simulink model "Autopilot_q_full_5may_new1"  (R2020a)
settings: Solver=ode4  StartTime=0.0  StopTime=300  FixedStep=0.01  RelTol=1e-3
undefined symbols (not defined in the file or in its folder): Aero_cofficients, Atmosphere_pert, Atmospheric_model, Counter_sensor_model, Earth, error_global, flags_global, Guidance_Flags_global, INT_global, param_guidance, Payload_data, Plane_state_mode_finish_catcher_ftr_mode, Plane_state_mode_finish_catcher_fw_mode, Plane_state_mode_finish_catcher_q_mode, Plane_state_mode_finish_catcher_rtr_mode, Plane_state_store, propulsion_model, propulsion_model_int, Structural_data, Thrust_data_store, time_global, WGS84, Wind_data, Wind_model_int, Wind_pert_factor
libraries: simulink x33, aerolibactuator x15, cstblocks x3, aerolibatmos2 x2, aerolibfltsims x1, aerolibtransform2 x1, shared6dof x1
(part 3 of 10)

== system Autopilot_q_full_5may_new1/AUTOPILOT /Autopilot Fixed wing mode/Roll controller ==
  stall_speed : Inport
  Plane_state : Inport  Port=2
  a_y_d : Inport  Port=3
  Aero_coffecients read3 : DataStoreRead  DataStoreName=Aero_cofficients  DataStoreElements=Aero_cofficients(:,:)
  Constant{6..11} (6 alike) : Constant
  Data Store Read : DataStoreRead  DataStoreName=Thrust_data_store  DataStoreElements=Thrust_data_store(:,:)
  Data Store Read1 : DataStoreRead  DataStoreName=param_guidance  DataStoreElements=param_guidance(:)
  Data Store Read13 : DataStoreRead  DataStoreName=propulsion_model  DataStoreElements=propulsion_model(:)
  Data Store Read15 : DataStoreRead  DataStoreName=Atmospheric_model
  Data Store Read2 : DataStoreRead  DataStoreName=Wind_data  DataStoreElements=Wind_data(:)
  Digital Clock : DigitalClock  SampleTime=0.01
  Gain{,1..3} (4 alike) : Gain  Gain=57.3
  MATLAB Function1 : MATLAB Function  TreatAsAtomicUnit=on
  MATLAB Function2 : MATLAB Function  TreatAsAtomicUnit=on
  PID Controller (2DOF) : simulink/Continuous/PID Controller (2DOF)  Controller=PID  Form=Parallel  TimeDomain=Discrete-time  UseExternalTs=off  SampleTime=0.01  IntegratorMethod=Forward Euler  FilterMethod=Forward Euler  ControllerParametersSource=internal  P=4.0  I=0.3  D=0  UseFilter=on  N=100  b=1  c=1  TunerSelectOption=Transfer Function Based (PID Tuner App)  InitialConditionSource=internal  InitialConditionForIntegrator=0  InitialConditionForFilter=0  DifferentiatorICPrevScaledInput=0  ExternalReset=none  TrackingMode=off  Kt=1  LimitOutput=off  UpperSaturationLimit=inf  LowerSaturationLimit=-inf  LinearizeAsGain=on  AntiWindupMode=none  Kb=1  POutMin=[]  POutMax=[]  IOutMin=[]  IOutMax=[]  DOutMin=[]  DOutMax=[]  NOutMin=[]  NOutMax=[]  bOutMin=[]  bOutMax=[]  cOutMin=[]  cOutMax=[]  SumOutMin=[]  SumOutMax=[]  SaturationOutMin=[]  SaturationOutMax=[]  PParamMin=[]  PParamMax=[]  IParamMin=[]  IParamMax=[]  DParamMin=[]  DParamMax=[]  NParamMin=[]  NParamMax=[]  bParamMin=[]  bParamMax=[]  cParamMin=[]  cParamMax=[]  KbParamMin=[]  KbParamMax=[]  KtParamMin=[]  KtParamMax=[]  KbOutMin=[]  KbOutMax=[]  KtOutMin=[]  KtOutMax=[]  IntegratorOutMin=[]  IntegratorOutMax=[]  FilterOutMin=[]  FilterOutMax=[]  SumI1OutMin=[]  SumI1OutMax=[]  SumI2OutMin=[]  SumI2OutMax=[]  SumI3OutMin=[]  SumI3OutMax=[]  SumI4OutMin=[]  SumI4OutMax=[]  SumDOutMin=[]  SumDOutMax=[]  Sum1OutMin=[]  Sum1OutMax=[]  Sum2OutMin=[]  Sum2OutMax=[]  Sum3OutMin=[]  Sum3OutMax=[]  DifferentiatorOutMin=[]  DifferentiatorOutMax=[]  FilterDiffOutCoefMin=[]  FilterDiffOutCoefMax=[]  ReciprocalOutMin=[]  ReciprocalOutMax=[]  SumDenOutMin=[]  SumDenOutMax=[]  SumNumOutMin=[]  SumNumOutMax=[]  DivideOutMin=[]  DivideOutMax=[]  UdiffTsProdOutMin=[]  UdiffTsProdOutMax=[]  NTsProdOutMin=[]  NTsProdOutMax=[]  UintegralTsProdOutMin=[]  UintegralTsProdOutMax=[]  UngainTsProdOutMin=[]  UngainTsProdOutMax=[]  IntegratorContinuousStateAttributes=''  IntegratorStateMustResolveToSignalObject=off  IntegratorRTWStateStorageClass=Auto  FilterContinuousStateAttributes=''  FilterStateMustResolveToSignalObject=off  FilterRTWStateStorageClass=Auto  ParallelPVariant=InternalParameters  IdealPVariant=Disabled  IVariant=InternalParameters  DVariant=InternalParameters  bVariant=InternalParameters  cVariant=InternalParameters  IntegratorVariant=Discrete  SatVariant=Disabled  AWVariant=Passthrough  PCopyVariant=Disabled  TRVariant=Disabled  FdbkBlocksVariant=Forward  IdealPFdbkVariant=Disabled  SatFdbkVariant=Disabled  DerivativeFilterVariant=ForwardEulerFilter  NVariant=InternalParameters  NCopyVariant=Disabled  FilterICVariant=InternalICsFilter  IntegratorICVariant=InternalICs  ExternalResetVariant=Disabled  TRSumVariant=Passthrough  SumFdbkVariant=Disabled  SumVariant=Sum_PID  TsampFilterVariant=InternalTs  TsampNgainVariant=Passthrough  TsampIntegralVariant=Passthrough
  PID Controller (2DOF)1 : simulink/Continuous/PID Controller (2DOF)  Controller=PID  Form=Parallel  TimeDomain=Discrete-time  UseExternalTs=off  SampleTime=0.01  IntegratorMethod=Forward Euler  FilterMethod=Forward Euler  ControllerParametersSource=internal  P=12.0  I=6.0  D=0  UseFilter=on  N=100  b=1  c=1  TunerSelectOption=Transfer Function Based (PID Tuner App)  InitialConditionSource=internal  InitialConditionForIntegrator=0  InitialConditionForFilter=0  DifferentiatorICPrevScaledInput=0  ExternalReset=none  TrackingMode=off  Kt=1  LimitOutput=off  UpperSaturationLimit=inf  LowerSaturationLimit=-inf  LinearizeAsGain=on  AntiWindupMode=none  Kb=1  POutMin=[]  POutMax=[]  IOutMin=[]  IOutMax=[]  DOutMin=[]  DOutMax=[]  NOutMin=[]  NOutMax=[]  bOutMin=[]  bOutMax=[]  cOutMin=[]  cOutMax=[]  SumOutMin=[]  SumOutMax=[]  SaturationOutMin=[]  SaturationOutMax=[]  PParamMin=[]  PParamMax=[]  IParamMin=[]  IParamMax=[]  DParamMin=[]  DParamMax=[]  NParamMin=[]  NParamMax=[]  bParamMin=[]  bParamMax=[]  cParamMin=[]  cParamMax=[]  KbParamMin=[]  KbParamMax=[]  KtParamMin=[]  KtParamMax=[]  KbOutMin=[]  KbOutMax=[]  KtOutMin=[]  KtOutMax=[]  IntegratorOutMin=[]  IntegratorOutMax=[]  FilterOutMin=[]  FilterOutMax=[]  SumI1OutMin=[]  SumI1OutMax=[]  SumI2OutMin=[]  SumI2OutMax=[]  SumI3OutMin=[]  SumI3OutMax=[]  SumI4OutMin=[]  SumI4OutMax=[]  SumDOutMin=[]  SumDOutMax=[]  Sum1OutMin=[]  Sum1OutMax=[]  Sum2OutMin=[]  Sum2OutMax=[]  Sum3OutMin=[]  Sum3OutMax=[]  DifferentiatorOutMin=[]  DifferentiatorOutMax=[]  FilterDiffOutCoefMin=[]  FilterDiffOutCoefMax=[]  ReciprocalOutMin=[]  ReciprocalOutMax=[]  SumDenOutMin=[]  SumDenOutMax=[]  SumNumOutMin=[]  SumNumOutMax=[]  DivideOutMin=[]  DivideOutMax=[]  UdiffTsProdOutMin=[]  UdiffTsProdOutMax=[]  NTsProdOutMin=[]  NTsProdOutMax=[]  UintegralTsProdOutMin=[]  UintegralTsProdOutMax=[]  UngainTsProdOutMin=[]  UngainTsProdOutMax=[]  IntegratorContinuousStateAttributes=''  IntegratorStateMustResolveToSignalObject=off  IntegratorRTWStateStorageClass=Auto  FilterContinuousStateAttributes=''  FilterStateMustResolveToSignalObject=off  FilterRTWStateStorageClass=Auto  ParallelPVariant=InternalParameters  IdealPVariant=Disabled  IVariant=InternalParameters  DVariant=InternalParameters  bVariant=InternalParameters  cVariant=InternalParameters  IntegratorVariant=Discrete  SatVariant=Disabled  AWVariant=Passthrough  PCopyVariant=Disabled  TRVariant=Disabled  FdbkBlocksVariant=Forward  IdealPFdbkVariant=Disabled  SatFdbkVariant=Disabled  DerivativeFilterVariant=ForwardEulerFilter  NVariant=InternalParameters  NCopyVariant=Disabled  FilterICVariant=InternalICsFilter  IntegratorICVariant=InternalICs  ExternalResetVariant=Disabled  TRSumVariant=Passthrough  SumFdbkVariant=Disabled  SumVariant=Sum_PID  TsampFilterVariant=InternalTs  TsampNgainVariant=Passthrough  TsampIntegralVariant=Passthrough
  Scope : Scope  NumInputPorts=2
  Scope1 : Scope  NumInputPorts=2
  Structure_data_read2 : DataStoreRead  DataStoreName=Structural_data  DataStoreElements=Structural_data(:,:)
  Terminator : Terminator
  mass : DataStoreRead  DataStoreName=Structural_data  DataStoreElements=Structural_data(1,1)
  p : DataStoreRead  DataStoreName=Plane_state_store  DataStoreElements=Plane_state_store(1,4)
  phi : DataStoreRead  DataStoreName=Plane_state_store  DataStoreElements=Plane_state_store(1,7)
  pqr,phi,theta,psi : DataStoreRead  DataStoreName=Plane_state_store  DataStoreElements=Plane_state_store(1,4:9)
  p_dot_d : Outport  VectorParamsAs1DForOutWhenUnconnected=off
  wires:
  p/1 -> Gain3/1, PID Controller (2DOF)1/2
  phi/1 -> PID Controller (2DOF)/2, Gain1/1
  pqr,phi,theta,psi/1 -> MATLAB Function2/1(angular_state)
  PID Controller (2DOF)/1 -> MATLAB Function2/2(phi_dot_d)
  mass/1 -> MATLAB Function1/3(mass)
  Data Store Read/1 -> MATLAB Function1/2(Thrust)
  Aero_coffecients read3/1 -> MATLAB Function1/5(aero_data)
  Digital Clock/1 -> MATLAB Function1/1(t)
  Structure_data_read2/1 -> MATLAB Function1/6(structure_data)
  MATLAB Function1/1(phi_d) -> PID Controller (2DOF)/1, Gain/1
  PID Controller (2DOF)1/1 -> p_dot_d/1
  a_y_d/1 -> MATLAB Function1/4(a_y_d)
  Plane_state/1 -> MATLAB Function1/7(Plane_state)
  Gain/1 -> Scope/1
  Gain1/1 -> Scope/2
  Gain2/1 -> Scope1/1
  Gain3/1 -> Scope1/2
  MATLAB Function2/1(p_d) -> Gain2/1, PID Controller (2DOF)1/1
  Data Store Read1/1 -> MATLAB Function1/8(param_guidance)
  stall_speed/1 -> Terminator/1
  Data Store Read2/1 -> MATLAB Function1/9(Wind_ned)
  Data Store Read13/1 -> MATLAB Function1/10(propulsion_data)
  Data Store Read15/1 -> MATLAB Function1/11(atmos_data)
  Constant6/1 -> MATLAB Function1/12(data2)
  Constant7/1 -> MATLAB Function1/13(data3)
  Constant8/1 -> MATLAB Function1/15(data4)
  Constant9/1 -> MATLAB Function1/14(data5)
  Constant10/1 -> MATLAB Function1/16(data6)
  Constant11/1 -> MATLAB Function1/17(data7)

== system Autopilot_q_full_5may_new1/AUTOPILOT /Autopilot Fixed wing mode/Trim setting ==
  "aero " : Inport
  "struct " : Inport  Port=2
  V_trim : Inport  Port=3
  Data Store Read11 : DataStoreRead  DataStoreName=propulsion_model  DataStoreElements=propulsion_model(:)
  Data Store Read14 : DataStoreRead  DataStoreName=Atmospheric_model
  MATLAB Function : MATLAB Function  TreatAsAtomicUnit=on
  alpha_trim : Outport  VectorParamsAs1DForOutWhenUnconnected=off
  beta_trim : Outport  Port=2  VectorParamsAs1DForOutWhenUnconnected=off
  delta_e_trim : Outport  Port=3  VectorParamsAs1DForOutWhenUnconnected=off
  delta_a_trim : Outport  Port=4  VectorParamsAs1DForOutWhenUnconnected=off
  delta_r_trim : Outport  Port=5  VectorParamsAs1DForOutWhenUnconnected=off
  Tx_trim : Outport  Port=6  VectorParamsAs1DForOutWhenUnconnected=off
  stall_speed : Outport  Port=7  VectorParamsAs1DForOutWhenUnconnected=off
  wires:
  "aero "/1 -> MATLAB Function/1(aero_data)
  "struct "/1 -> MATLAB Function/2(structure_data)
  V_trim/1 -> MATLAB Function/3(V_trim)
  MATLAB Function/1(alpha_trim) -> alpha_trim/1
  MATLAB Function/2(beta_trim) -> beta_trim/1
  MATLAB Function/3(delta_e_trim) -> delta_e_trim/1
  MATLAB Function/4(delta_a_trim) -> delta_a_trim/1
  MATLAB Function/5(delta_r_trim) -> delta_r_trim/1
  MATLAB Function/6(Tx_trim) -> Tx_trim/1
  MATLAB Function/7(stall_speed) -> stall_speed/1
  Data Store Read11/1 -> MATLAB Function/4(propulsion_data)
  Data Store Read14/1 -> MATLAB Function/5(atmos_data)

== system Autopilot_q_full_5may_new1/AUTOPILOT /Autopilot Fixed wing mode/beta controller ==
  acc_d : Inport
  Plane_state : Inport  Port=2
  stall_speed : Inport  Port=3
  Aero_coffecients read2 : DataStoreRead  DataStoreName=Aero_cofficients  DataStoreElements=Aero_cofficients(:,:)
  Constant{6..11} (6 alike) : Constant
  Data Store Read : DataStoreRead  DataStoreName=Wind_data  DataStoreElements=Wind_data(:)
  Data Store Read13 : DataStoreRead  DataStoreName=propulsion_model  DataStoreElements=propulsion_model(:)
  Data Store Read15 : DataStoreRead  DataStoreName=Atmospheric_model
  Data Store Read3 : DataStoreRead  DataStoreName=Thrust_data_store  DataStoreElements=Thrust_data_store(:,:)
  Gain{,1..3} (4 alike) : Gain  Gain=57.3
  PID Controller (2DOF)1 : simulink/Continuous/PID Controller (2DOF)  Controller=PID  TimeDomain=Discrete-time  SampleTime=0.01  IntegratorMethod=Forward Euler  FilterMethod=Forward Euler  Form=Parallel  UseFilter=on  ControllerParametersSource=internal  P=1.8  I=0.5  D=0  N=100  b=1  c=1  InitialConditionSource=internal  InitialConditionForIntegrator=0  InitialConditionForFilter=0  ExternalReset=none  LimitOutput=off  UpperSaturationLimit=inf  LowerSaturationLimit=-inf  LinearizeAsGain=on  AntiWindupMode=none  Kb=1  TrackingMode=off  Kt=1  PParamMin=[]  PParamMax=[]  IParamMin=[]  IParamMax=[]  DParamMin=[]  DParamMax=[]  NParamMin=[]  NParamMax=[]  bParamMin=[]  bParamMax=[]  cParamMin=[]  cParamMax=[]  KbParamMin=[]  KbParamMax=[]  KtParamMin=[]  KtParamMax=[]  POutMin=[]  POutMax=[]  IOutMin=[]  IOutMax=[]  DOutMin=[]  DOutMax=[]  NOutMin=[]  NOutMax=[]  bOutMin=[]  bOutMax=[]  cOutMin=[]  cOutMax=[]  KbOutMin=[]  KbOutMax=[]  KtOutMin=[]  KtOutMax=[]  IntegratorOutMin=[]  IntegratorOutMax=[]  FilterOutMin=[]  FilterOutMax=[]  SumOutMin=[]  SumOutMax=[]  Sum1OutMin=[]  Sum1OutMax=[]  Sum2OutMin=[]  Sum2OutMax=[]  Sum3OutMin=[]  Sum3OutMax=[]  SumI1OutMin=[]  SumI1OutMax=[]  SumI2OutMin=[]  SumI2OutMax=[]  SumI3OutMin=[]  SumI3OutMax=[]  SumDOutMin=[]  SumDOutMax=[]  SaturationOutMin=[]  SaturationOutMax=[]  IntegratorContinuousStateAttributes=''  IntegratorStateMustResolveToSignalObject=off  IntegratorRTWStateStorageClass=Auto  FilterContinuousStateAttributes=''  FilterStateMustResolveToSignalObject=off  FilterRTWStateStorageClass=Auto  DifferentiatorICPrevScaledInput=0  DifferentiatorOutMin=[]  DifferentiatorOutMax=[]  FilterDiffOutCoefMin=[]  FilterDiffOutCoefMax=[]  SumDenOutMin=[]  SumDenOutMax=[]  SumNumOutMin=[]  SumNumOutMax=[]  ReciprocalOutMin=[]  ReciprocalOutMax=[]  DivideOutMin=[]  DivideOutMax=[]  TunerSelectOption=Transfer Function Based (PID Tuner App)
  PID Controller (2DOF)2 : simulink/Continuous/PID Controller (2DOF)  Controller=PID  TimeDomain=Discrete-time  SampleTime=0.01  IntegratorMethod=Forward Euler  FilterMethod=Forward Euler  Form=Parallel  UseFilter=on  ControllerParametersSource=internal  P=0.66  I=0  D=0  N=100  b=1  c=1  InitialConditionSource=internal  InitialConditionForIntegrator=0  InitialConditionForFilter=0  ExternalReset=none  LimitOutput=off  UpperSaturationLimit=inf  LowerSaturationLimit=-inf  LinearizeAsGain=on  AntiWindupMode=none  Kb=1  TrackingMode=off  Kt=1  PParamMin=[]  PParamMax=[]  IParamMin=[]  IParamMax=[]  DParamMin=[]  DParamMax=[]  NParamMin=[]  NParamMax=[]  bParamMin=[]  bParamMax=[]  cParamMin=[]  cParamMax=[]  KbParamMin=[]  KbParamMax=[]  KtParamMin=[]  KtParamMax=[]  POutMin=[]  POutMax=[]  IOutMin=[]  IOutMax=[]  DOutMin=[]  DOutMax=[]  NOutMin=[]  NOutMax=[]  bOutMin=[]  bOutMax=[]  cOutMin=[]  cOutMax=[]  KbOutMin=[]  KbOutMax=[]  KtOutMin=[]  KtOutMax=[]  IntegratorOutMin=[]  IntegratorOutMax=[]  FilterOutMin=[]  FilterOutMax=[]  SumOutMin=[]  SumOutMax=[]  Sum1OutMin=[]  Sum1OutMax=[]  Sum2OutMin=[]  Sum2OutMax=[]  Sum3OutMin=[]  Sum3OutMax=[]  SumI1OutMin=[]  SumI1OutMax=[]  SumI2OutMin=[]  SumI2OutMax=[]  SumI3OutMin=[]  SumI3OutMax=[]  SumDOutMin=[]  SumDOutMax=[]  SaturationOutMin=[]  SaturationOutMax=[]  IntegratorContinuousStateAttributes=''  IntegratorStateMustResolveToSignalObject=off  IntegratorRTWStateStorageClass=Auto  FilterContinuousStateAttributes=''  FilterStateMustResolveToSignalObject=off  FilterRTWStateStorageClass=Auto  DifferentiatorICPrevScaledInput=0  DifferentiatorOutMin=[]  DifferentiatorOutMax=[]  FilterDiffOutCoefMin=[]  FilterDiffOutCoefMax=[]  SumDenOutMin=[]  SumDenOutMax=[]  SumNumOutMin=[]  SumNumOutMax=[]  ReciprocalOutMin=[]  ReciprocalOutMax=[]  DivideOutMin=[]  DivideOutMax=[]  TunerSelectOption=Transfer Function Based (PID Tuner App)
  Scope : Scope  NumInputPorts=2
  Scope1 : Scope  NumInputPorts=2
  Structure_data_read1 : DataStoreRead  DataStoreName=Structural_data  DataStoreElements=Structural_data(:,:)
  beta_controller : MATLAB Function  TreatAsAtomicUnit=on
  r_dot_d : Outport  VectorParamsAs1DForOutWhenUnconnected=off
  wires:
  Aero_coffecients read2/1 -> beta_controller/3(aero_data)
  Structure_data_read1/1 -> beta_controller/4(structure_data)
  Data Store Read3/1 -> beta_controller/5(Thrust)
  beta_controller/1(beta_d) -> Gain/1, PID Controller (2DOF)2/1
  Plane_state/1 -> beta_controller/2(Plane_state)
  acc_d/1 -> beta_controller/1(acc_d)
  beta_controller/2(beta) -> PID Controller (2DOF)2/2, Gain1/1
  PID Controller (2DOF)1/1 -> r_dot_d/1
  stall_speed/1 -> beta_controller/6(V_stall)
  Gain/1 -> Scope/1
  Gain1/1 -> Scope/2
  Gain2/1 -> Scope1/1
  beta_controller/3(r) -> PID Controller (2DOF)1/2, Gain3/1
  Gain3/1 -> Scope1/2
  PID Controller (2DOF)2/1 -> Gain2/1, PID Controller (2DOF)1/1
  Data Store Read/1 -> beta_controller/7(Wind_ned)
  Data Store Read13/1 -> beta_controller/8(propulsion_data)
  Data Store Read15/1 -> beta_controller/9(atmos_data)
  Constant6/1 -> beta_controller/10(data2)
  Constant7/1 -> beta_controller/11(data3)
  Constant8/1 -> beta_controller/12(data4)
  Constant9/1 -> beta_controller/13(data5)
  Constant10/1 -> beta_controller/14(data6)
  Constant11/1 -> beta_controller/15(data7)

== system Autopilot_q_full_5may_new1/AUTOPILOT /Autopilot Quad mode/Heading Controller ==
  Data Store Read4 : DataStoreRead  DataStoreName=Plane_state_mode_finish_catcher_rtr_mode  SampleTime=0.01  DataStoreElements=Plane_state_mode_finish_catcher_rtr_mode(9)
  Demux1 : Demux  Outputs=2
  Digital Clock : DigitalClock  SampleTime=0.01
  MATLAB Function : MATLAB Function  TreatAsAtomicUnit=on
  MATLAB Function5 : MATLAB Function  TreatAsAtomicUnit=on
  MATLAB Function6 : MATLAB Function  TreatAsAtomicUnit=on
  PID Controller : simulink/Continuous/PID Controller  Controller=PID  Form=Parallel  TimeDomain=Discrete-time  UseExternalTs=off  SampleTime=0.01  IntegratorMethod=Forward Euler  FilterMethod=Forward Euler  ControllerParametersSource=internal  P=0.66  I=0  D=0  UseFilter=on  N=100  TunerSelectOption=Transfer Function Based (PID Tuner App)  InitialConditionSource=internal  InitialConditionForIntegrator=0  InitialConditionForFilter=0  DifferentiatorICPrevScaledInput=0  ExternalReset=none  TrackingMode=off  Kt=1  LimitOutput=off  UpperSaturationLimit=inf  LowerSaturationLimit=-inf  LinearizeAsGain=on  AntiWindupMode=none  Kb=1  POutMin=[]  POutMax=[]  IOutMin=[]  IOutMax=[]  DOutMin=[]  DOutMax=[]  NOutMin=[]  NOutMax=[]  SumOutMin=[]  SumOutMax=[]  SaturationOutMin=[]  SaturationOutMax=[]  PParamMin=[]  PParamMax=[]  IParamMin=[]  IParamMax=[]  DParamMin=[]  DParamMax=[]  NParamMin=[]  NParamMax=[]  KbParamMin=[]  KbParamMax=[]  KtParamMin=[]  KtParamMax=[]  KbOutMin=[]  KbOutMax=[]  KtOutMin=[]  KtOutMax=[]  IntegratorOutMin=[]  IntegratorOutMax=[]  FilterOutMin=[]  FilterOutMax=[]  SumI1OutMin=[]  SumI1OutMax=[]  SumI2OutMin=[]  SumI2OutMax=[]  SumI3OutMin=[]  SumI3OutMax=[]  SumI4OutMin=[]  SumI4OutMax=[]  SumDOutMin=[]  SumDOutMax=[]  DifferentiatorOutMin=[]  DifferentiatorOutMax=[]  FilterDiffOutCoefMin=[]  FilterDiffOutCoefMax=[]  ReciprocalOutMin=[]  ReciprocalOutMax=[]  SumDenOutMin=[]  SumDenOutMax=[]  SumNumOutMin=[]  SumNumOutMax=[]  DivideOutMin=[]  DivideOutMax=[]  UdiffTsProdOutMin=[]  UdiffTsProdOutMax=[]  NTsProdOutMin=[]  NTsProdOutMax=[]  UintegralTsProdOutMin=[]  UintegralTsProdOutMax=[]  UngainTsProdOutMin=[]  UngainTsProdOutMax=[]  IntegratorContinuousStateAttributes=''  IntegratorStateMustResolveToSignalObject=off  IntegratorRTWStateStorageClass=Auto  FilterContinuousStateAttributes=''  FilterStateMustResolveToSignalObject=off  FilterRTWStateStorageClass=Auto  ParallelPVariant=InternalParameters  IdealPVariant=Disabled  IVariant=InternalParameters  DVariant=InternalParameters  IntegratorVariant=Discrete  SatVariant=Disabled  AWVariant=Passthrough  PCopyVariant=Disabled  TRVariant=Disabled  FdbkBlocksVariant=Forward  IdealPFdbkVariant=Disabled  SatFdbkVariant=Disabled  DerivativeFilterVariant=ForwardEulerFilter  NVariant=InternalParameters  NCopyVariant=Disabled  FilterICVariant=InternalICsFilter  IntegratorICVariant=InternalICs  ExternalResetVariant=Disabled  TRSumVariant=Passthrough  SumFdbkVariant=Disabled  SumVariant=Sum_PID  TsampFilterVariant=InternalTs  TsampNgainVariant=Passthrough  TsampIntegralVariant=Passthrough
  PID Controller (2DOF)5 : simulink/Continuous/PID Controller (2DOF)  Controller=PID  Form=Parallel  TimeDomain=Discrete-time  UseExternalTs=off  SampleTime=0.01  IntegratorMethod=Forward Euler  FilterMethod=Forward Euler  ControllerParametersSource=internal  P=2  I=0.5  D=0  UseFilter=on  N=100  b=1  c=1  TunerSelectOption=Transfer Function Based (PID Tuner App)  InitialConditionSource=internal  InitialConditionForIntegrator=0  InitialConditionForFilter=0  DifferentiatorICPrevScaledInput=0  ExternalReset=none  TrackingMode=off  Kt=1  LimitOutput=off  UpperSaturationLimit=inf  LowerSaturationLimit=-inf  LinearizeAsGain=on  AntiWindupMode=none  Kb=1  POutMin=[]  POutMax=[]  IOutMin=[]  IOutMax=[]  DOutMin=[]  DOutMax=[]  NOutMin=[]  NOutMax=[]  bOutMin=[]  bOutMax=[]  cOutMin=[]  cOutMax=[]  SumOutMin=[]  SumOutMax=[]  SaturationOutMin=[]  SaturationOutMax=[]  PParamMin=[]  PParamMax=[]  IParamMin=[]  IParamMax=[]  DParamMin=[]  DParamMax=[]  NParamMin=[]  NParamMax=[]  bParamMin=[]  bParamMax=[]  cParamMin=[]  cParamMax=[]  KbParamMin=[]  KbParamMax=[]  KtParamMin=[]  KtParamMax=[]  KbOutMin=[]  KbOutMax=[]  KtOutMin=[]  KtOutMax=[]  IntegratorOutMin=[]  IntegratorOutMax=[]  FilterOutMin=[]  FilterOutMax=[]  SumI1OutMin=[]  SumI1OutMax=[]  SumI2OutMin=[]  SumI2OutMax=[]  SumI3OutMin=[]  SumI3OutMax=[]  SumI4OutMin=[]  SumI4OutMax=[]  SumDOutMin=[]  SumDOutMax=[]  Sum1OutMin=[]  Sum1OutMax=[]  Sum2OutMin=[]  Sum2OutMax=[]  Sum3OutMin=[]  Sum3OutMax=[]  DifferentiatorOutMin=[]  DifferentiatorOutMax=[]  FilterDiffOutCoefMin=[]  FilterDiffOutCoefMax=[]  ReciprocalOutMin=[]  ReciprocalOutMax=[]  SumDenOutMin=[]  SumDenOutMax=[]  SumNumOutMin=[]  SumNumOutMax=[]  DivideOutMin=[]  DivideOutMax=[]  UdiffTsProdOutMin=[]  UdiffTsProdOutMax=[]  NTsProdOutMin=[]  NTsProdOutMax=[]  UintegralTsProdOutMin=[]  UintegralTsProdOutMax=[]  UngainTsProdOutMin=[]  UngainTsProdOutMax=[]  IntegratorContinuousStateAttributes=''  IntegratorStateMustResolveToSignalObject=off  IntegratorRTWStateStorageClass=Auto  FilterContinuousStateAttributes=''  FilterStateMustResolveToSignalObject=off  FilterRTWStateStorageClass=Auto  ParallelPVariant=InternalParameters  IdealPVariant=Disabled  IVariant=InternalParameters  DVariant=InternalParameters  bVariant=InternalParameters  cVariant=InternalParameters  IntegratorVariant=Discrete  SatVariant=Disabled  AWVariant=Passthrough  PCopyVariant=Disabled  TRVariant=Disabled  FdbkBlocksVariant=Forward  IdealPFdbkVariant=Disabled  SatFdbkVariant=Disabled  DerivativeFilterVariant=ForwardEulerFilter  NVariant=InternalParameters  NCopyVariant=Disabled  FilterICVariant=InternalICsFilter  IntegratorICVariant=InternalICs  ExternalResetVariant=Disabled  TRSumVariant=Passthrough  SumFdbkVariant=Disabled  SumVariant=Sum_PID  TsampFilterVariant=InternalTs  TsampNgainVariant=Passthrough  TsampIntegralVariant=Passthrough
  p,q,r,phi,theta,psi : DataStoreRead  DataStoreName=Plane_state_store  DataStoreElements=Plane_state_store(1,4:9)
  psi : DataStoreRead  DataStoreName=Plane_state_store  DataStoreElements=Plane_state_store(1,9)
  r : DataStoreRead  DataStoreName=Plane_state_store  DataStoreElements=Plane_state_store(1,6)
  u,v : DataStoreRead  DataStoreName=Plane_state_store  SampleTime=0.01  DataStoreElements=Plane_state_store(1,1:2)
  Out1 : Outport  VectorParamsAs1DForOutWhenUnconnected=off
  wires:
  MATLAB Function5/1(psi_d) -> MATLAB Function/1(psi_d)
  u,v/1 -> Demux1/1
  Data Store Read4/1 -> MATLAB Function5/4("psi_d ")
  Digital Clock/1 -> MATLAB Function5/1(t)
  Demux1/1 -> MATLAB Function5/2(u)
  p,q,r,phi,theta,psi/1 -> MATLAB Function6/1(angular_state)
  psi/1 -> MATLAB Function/2(psi)
  MATLAB Function6/1(r_d) -> PID Controller (2DOF)5/1
  PID Controller/1 -> MATLAB Function6/2(psi_dot_d)
  MATLAB Function/1(psi_error) -> PID Controller/1
  Demux1/2 -> MATLAB Function5/3(v)
  PID Controller (2DOF)5/1 -> Out1/1
  r/1 -> PID Controller (2DOF)5/2

== system Autopilot_q_full_5may_new1/AUTOPILOT /Autopilot Quad mode/Pitch Controller ==
  a_x_d : Inport
  Data Store Read1 : DataStoreRead  DataStoreName=Thrust_data_store
  Digital Clock : DigitalClock  SampleTime=0.01
  MATLAB Function3 : MATLAB Function  TreatAsAtomicUnit=on
  MATLAB Function4 : MATLAB Function  TreatAsAtomicUnit=on
  PID Controller (2DOF)2 : simulink/Continuous/PID Controller (2DOF)  Controller=PID  Form=Parallel  TimeDomain=Discrete-time  UseExternalTs=off  SampleTime=0.01  IntegratorMethod=Forward Euler  FilterMethod=Forward Euler  ControllerParametersSource=internal  P=4.0  I=0  D=0  UseFilter=on  N=100  b=1  c=1  TunerSelectOption=Transfer Function Based (PID Tuner App)  InitialConditionSource=internal  InitialConditionForIntegrator=0  InitialConditionForFilter=0  DifferentiatorICPrevScaledInput=0  ExternalReset=none  TrackingMode=off  Kt=1  LimitOutput=off  UpperSaturationLimit=inf  LowerSaturationLimit=-inf  LinearizeAsGain=on  AntiWindupMode=none  Kb=1  POutMin=[]  POutMax=[]  IOutMin=[]  IOutMax=[]  DOutMin=[]  DOutMax=[]  NOutMin=[]  NOutMax=[]  bOutMin=[]  bOutMax=[]  cOutMin=[]  cOutMax=[]  SumOutMin=[]  SumOutMax=[]  SaturationOutMin=[]  SaturationOutMax=[]  PParamMin=[]  PParamMax=[]  IParamMin=[]  IParamMax=[]  DParamMin=[]  DParamMax=[]  NParamMin=[]  NParamMax=[]  bParamMin=[]  bParamMax=[]  cParamMin=[]  cParamMax=[]  KbParamMin=[]  KbParamMax=[]  KtParamMin=[]  KtParamMax=[]  KbOutMin=[]  KbOutMax=[]  KtOutMin=[]  KtOutMax=[]  IntegratorOutMin=[]  IntegratorOutMax=[]  FilterOutMin=[]  FilterOutMax=[]  SumI1OutMin=[]  SumI1OutMax=[]  SumI2OutMin=[]  SumI2OutMax=[]  SumI3OutMin=[]  SumI3OutMax=[]  SumI4OutMin=[]  SumI4OutMax=[]  SumDOutMin=[]  SumDOutMax=[]  Sum1OutMin=[]  Sum1OutMax=[]  Sum2OutMin=[]  Sum2OutMax=[]  Sum3OutMin=[]  Sum3OutMax=[]  DifferentiatorOutMin=[]  DifferentiatorOutMax=[]  FilterDiffOutCoefMin=[]  FilterDiffOutCoefMax=[]  ReciprocalOutMin=[]  ReciprocalOutMax=[]  SumDenOutMin=[]  SumDenOutMax=[]  SumNumOutMin=[]  SumNumOutMax=[]  DivideOutMin=[]  DivideOutMax=[]  UdiffTsProdOutMin=[]  UdiffTsProdOutMax=[]  NTsProdOutMin=[]  NTsProdOutMax=[]  UintegralTsProdOutMin=[]  UintegralTsProdOutMax=[]  UngainTsProdOutMin=[]  UngainTsProdOutMax=[]  IntegratorContinuousStateAttributes=''  IntegratorStateMustResolveToSignalObject=off  IntegratorRTWStateStorageClass=Auto  FilterContinuousStateAttributes=''  FilterStateMustResolveToSignalObject=off  FilterRTWStateStorageClass=Auto  ParallelPVariant=InternalParameters  IdealPVariant=Disabled  IVariant=InternalParameters  DVariant=InternalParameters  bVariant=InternalParameters  cVariant=InternalParameters  IntegratorVariant=Discrete  SatVariant=Disabled  AWVariant=Passthrough  PCopyVariant=Disabled  TRVariant=Disabled  FdbkBlocksVariant=Forward  IdealPFdbkVariant=Disabled  SatFdbkVariant=Disabled  DerivativeFilterVariant=ForwardEulerFilter  NVariant=InternalParameters  NCopyVariant=Disabled  FilterICVariant=InternalICsFilter  IntegratorICVariant=InternalICs  ExternalResetVariant=Disabled  TRSumVariant=Passthrough  SumFdbkVariant=Disabled  SumVariant=Sum_PID  TsampFilterVariant=InternalTs  TsampNgainVariant=Passthrough  TsampIntegralVariant=Passthrough
  PID Controller (2DOF)3 : simulink/Continuous/PID Controller (2DOF)  Controller=PID  Form=Parallel  TimeDomain=Discrete-time  UseExternalTs=off  SampleTime=0.01  IntegratorMethod=Forward Euler  FilterMethod=Forward Euler  ControllerParametersSource=internal  P=12.0  I=0.1  D=0  UseFilter=on  N=100  b=1  c=1  TunerSelectOption=Transfer Function Based (PID Tuner App)  InitialConditionSource=internal  InitialConditionForIntegrator=0  InitialConditionForFilter=0  DifferentiatorICPrevScaledInput=0  ExternalReset=none  TrackingMode=off  Kt=1  LimitOutput=off  UpperSaturationLimit=inf  LowerSaturationLimit=-inf  LinearizeAsGain=on  AntiWindupMode=none  Kb=1  POutMin=[]  POutMax=[]  IOutMin=[]  IOutMax=[]  DOutMin=[]  DOutMax=[]  NOutMin=[]  NOutMax=[]  bOutMin=[]  bOutMax=[]  cOutMin=[]  cOutMax=[]  SumOutMin=[]  SumOutMax=[]  SaturationOutMin=[]  SaturationOutMax=[]  PParamMin=[]  PParamMax=[]  IParamMin=[]  IParamMax=[]  DParamMin=[]  DParamMax=[]  NParamMin=[]  NParamMax=[]  bParamMin=[]  bParamMax=[]  cParamMin=[]  cParamMax=[]  KbParamMin=[]  KbParamMax=[]  KtParamMin=[]  KtParamMax=[]  KbOutMin=[]  KbOutMax=[]  KtOutMin=[]  KtOutMax=[]  IntegratorOutMin=[]  IntegratorOutMax=[]  FilterOutMin=[]  FilterOutMax=[]  SumI1OutMin=[]  SumI1OutMax=[]  SumI2OutMin=[]  SumI2OutMax=[]  SumI3OutMin=[]  SumI3OutMax=[]  SumI4OutMin=[]  SumI4OutMax=[]  SumDOutMin=[]  SumDOutMax=[]  Sum1OutMin=[]  Sum1OutMax=[]  Sum2OutMin=[]  Sum2OutMax=[]  Sum3OutMin=[]  Sum3OutMax=[]  DifferentiatorOutMin=[]  DifferentiatorOutMax=[]  FilterDiffOutCoefMin=[]  FilterDiffOutCoefMax=[]  ReciprocalOutMin=[]  ReciprocalOutMax=[]  SumDenOutMin=[]  SumDenOutMax=[]  SumNumOutMin=[]  SumNumOutMax=[]  DivideOutMin=[]  DivideOutMax=[]  UdiffTsProdOutMin=[]  UdiffTsProdOutMax=[]  NTsProdOutMin=[]  NTsProdOutMax=[]  UintegralTsProdOutMin=[]  UintegralTsProdOutMax=[]  UngainTsProdOutMin=[]  UngainTsProdOutMax=[]  IntegratorContinuousStateAttributes=''  IntegratorStateMustResolveToSignalObject=off  IntegratorRTWStateStorageClass=Auto  FilterContinuousStateAttributes=''  FilterStateMustResolveToSignalObject=off  FilterRTWStateStorageClass=Auto  ParallelPVariant=InternalParameters  IdealPVariant=Disabled  IVariant=InternalParameters  DVariant=InternalParameters  bVariant=InternalParameters  cVariant=InternalParameters  IntegratorVariant=Discrete  SatVariant=Disabled  AWVariant=Passthrough  PCopyVariant=Disabled  TRVariant=Disabled  FdbkBlocksVariant=Forward  IdealPFdbkVariant=Disabled  SatFdbkVariant=Disabled  DerivativeFilterVariant=ForwardEulerFilter  NVariant=InternalParameters  NCopyVariant=Disabled  FilterICVariant=InternalICsFilter  IntegratorICVariant=InternalICs  ExternalResetVariant=Disabled  TRSumVariant=Passthrough  SumFdbkVariant=Disabled  SumVariant=Sum_PID  TsampFilterVariant=InternalTs  TsampNgainVariant=Passthrough  TsampIntegralVariant=Passthrough
  mass1 : DataStoreRead  DataStoreName=Structural_data  DataStoreElements=Structural_data(1,1)
  p,q,r,phi,theta,psi : DataStoreRead  DataStoreName=Plane_state_store  DataStoreElements=Plane_state_store(1,4:9)
  "q " : DataStoreRead  DataStoreName=Plane_state_store  DataStoreElements=Plane_state_store(1,5)
  theta : DataStoreRead  DataStoreName=Plane_state_store  DataStoreElements=Plane_state_store(1,8)
  Out1 : Outport  VectorParamsAs1DForOutWhenUnconnected=off
  wires:
  "q "/1 -> PID Controller (2DOF)3/2
  Digital Clock/1 -> MATLAB Function3/1(t)
  Data Store Read1/1 -> MATLAB Function3/2(TT)
  PID Controller (2DOF)2/1 -> MATLAB Function4/2(theta_dot_d)
  MATLAB Function4/1(q_d) -> PID Controller (2DOF)3/1
  p,q,r,phi,theta,psi/1 -> MATLAB Function4/1(angular_state)
  theta/1 -> PID Controller (2DOF)2/2
  MATLAB Function3/1(theta_d) -> PID Controller (2DOF)2/1
  mass1/1 -> MATLAB Function3/3(mass)
  a_x_d/1 -> MATLAB Function3/4(a_x_d)
  PID Controller (2DOF)3/1 -> Out1/1

== system Autopilot_q_full_5may_new1/AUTOPILOT /Autopilot Quad mode/Roll Controller ==
  a_y_d : Inport
  Data Store Read : DataStoreRead  DataStoreName=Thrust_data_store
  Digital Clock : DigitalClock  SampleTime=0.01
  MATLAB Function1 : MATLAB Function  TreatAsAtomicUnit=on
  MATLAB Function2 : MATLAB Function  TreatAsAtomicUnit=on
  PID Controller (2DOF) : simulink/Continuous/PID Controller (2DOF)  Controller=PID  Form=Parallel  TimeDomain=Discrete-time  UseExternalTs=off  SampleTime=0.01  IntegratorMethod=Forward Euler  FilterMethod=Forward Euler  ControllerParametersSource=internal  P=4.0  I=0  D=0  UseFilter=on  N=100  b=1  c=1  TunerSelectOption=Transfer Function Based (PID Tuner App)  InitialConditionSource=internal  InitialConditionForIntegrator=0  InitialConditionForFilter=0  DifferentiatorICPrevScaledInput=0  ExternalReset=none  TrackingMode=off  Kt=1  LimitOutput=off  UpperSaturationLimit=inf  LowerSaturationLimit=-inf  LinearizeAsGain=on  AntiWindupMode=none  Kb=1  POutMin=[]  POutMax=[]  IOutMin=[]  IOutMax=[]  DOutMin=[]  DOutMax=[]  NOutMin=[]  NOutMax=[]  bOutMin=[]  bOutMax=[]  cOutMin=[]  cOutMax=[]  SumOutMin=[]  SumOutMax=[]  SaturationOutMin=[]  SaturationOutMax=[]  PParamMin=[]  PParamMax=[]  IParamMin=[]  IParamMax=[]  DParamMin=[]  DParamMax=[]  NParamMin=[]  NParamMax=[]  bParamMin=[]  bParamMax=[]  cParamMin=[]  cParamMax=[]  KbParamMin=[]  KbParamMax=[]  KtParamMin=[]  KtParamMax=[]  KbOutMin=[]  KbOutMax=[]  KtOutMin=[]  KtOutMax=[]  IntegratorOutMin=[]  IntegratorOutMax=[]  FilterOutMin=[]  FilterOutMax=[]  SumI1OutMin=[]  SumI1OutMax=[]  SumI2OutMin=[]  SumI2OutMax=[]  SumI3OutMin=[]  SumI3OutMax=[]  SumI4OutMin=[]  SumI4OutMax=[]  SumDOutMin=[]  SumDOutMax=[]  Sum1OutMin=[]  Sum1OutMax=[]  Sum2OutMin=[]  Sum2OutMax=[]  Sum3OutMin=[]  Sum3OutMax=[]  DifferentiatorOutMin=[]  DifferentiatorOutMax=[]  FilterDiffOutCoefMin=[]  FilterDiffOutCoefMax=[]  ReciprocalOutMin=[]  ReciprocalOutMax=[]  SumDenOutMin=[]  SumDenOutMax=[]  SumNumOutMin=[]  SumNumOutMax=[]  DivideOutMin=[]  DivideOutMax=[]  UdiffTsProdOutMin=[]  UdiffTsProdOutMax=[]  NTsProdOutMin=[]  NTsProdOutMax=[]  UintegralTsProdOutMin=[]  UintegralTsProdOutMax=[]  UngainTsProdOutMin=[]  UngainTsProdOutMax=[]  IntegratorContinuousStateAttributes=''  IntegratorStateMustResolveToSignalObject=off  IntegratorRTWStateStorageClass=Auto  FilterContinuousStateAttributes=''  FilterStateMustResolveToSignalObject=off  FilterRTWStateStorageClass=Auto  ParallelPVariant=InternalParameters  IdealPVariant=Disabled  IVariant=InternalParameters  DVariant=InternalParameters  bVariant=InternalParameters  cVariant=InternalParameters  IntegratorVariant=Discrete  SatVariant=Disabled  AWVariant=Passthrough  PCopyVariant=Disabled  TRVariant=Disabled  FdbkBlocksVariant=Forward  IdealPFdbkVariant=Disabled  SatFdbkVariant=Disabled  DerivativeFilterVariant=ForwardEulerFilter  NVariant=InternalParameters  NCopyVariant=Disabled  FilterICVariant=InternalICsFilter  IntegratorICVariant=InternalICs  ExternalResetVariant=Disabled  TRSumVariant=Passthrough  SumFdbkVariant=Disabled  SumVariant=Sum_PID  TsampFilterVariant=InternalTs  TsampNgainVariant=Passthrough  TsampIntegralVariant=Passthrough
  PID Controller (2DOF)1 : simulink/Continuous/PID Controller (2DOF)  Controller=PID  Form=Parallel  TimeDomain=Discrete-time  UseExternalTs=off  SampleTime=0.01  IntegratorMethod=Forward Euler  FilterMethod=Forward Euler  ControllerParametersSource=internal  P=12.0  I=0.1  D=0  UseFilter=on  N=100  b=1  c=1  TunerSelectOption=Transfer Function Based (PID Tuner App)  InitialConditionSource=internal  InitialConditionForIntegrator=0  InitialConditionForFilter=0  DifferentiatorICPrevScaledInput=0  ExternalReset=none  TrackingMode=off  Kt=1  LimitOutput=off  UpperSaturationLimit=inf  LowerSaturationLimit=-inf  LinearizeAsGain=on  AntiWindupMode=none  Kb=1  POutMin=[]  POutMax=[]  IOutMin=[]  IOutMax=[]  DOutMin=[]  DOutMax=[]  NOutMin=[]  NOutMax=[]  bOutMin=[]  bOutMax=[]  cOutMin=[]  cOutMax=[]  SumOutMin=[]  SumOutMax=[]  SaturationOutMin=[]  SaturationOutMax=[]  PParamMin=[]  PParamMax=[]  IParamMin=[]  IParamMax=[]  DParamMin=[]  DParamMax=[]  NParamMin=[]  NParamMax=[]  bParamMin=[]  bParamMax=[]  cParamMin=[]  cParamMax=[]  KbParamMin=[]  KbParamMax=[]  KtParamMin=[]  KtParamMax=[]  KbOutMin=[]  KbOutMax=[]  KtOutMin=[]  KtOutMax=[]  IntegratorOutMin=[]  IntegratorOutMax=[]  FilterOutMin=[]  FilterOutMax=[]  SumI1OutMin=[]  SumI1OutMax=[]  SumI2OutMin=[]  SumI2OutMax=[]  SumI3OutMin=[]  SumI3OutMax=[]  SumI4OutMin=[]  SumI4OutMax=[]  SumDOutMin=[]  SumDOutMax=[]  Sum1OutMin=[]  Sum1OutMax=[]  Sum2OutMin=[]  Sum2OutMax=[]  Sum3OutMin=[]  Sum3OutMax=[]  DifferentiatorOutMin=[]  DifferentiatorOutMax=[]  FilterDiffOutCoefMin=[]  FilterDiffOutCoefMax=[]  ReciprocalOutMin=[]  ReciprocalOutMax=[]  SumDenOutMin=[]  SumDenOutMax=[]  SumNumOutMin=[]  SumNumOutMax=[]  DivideOutMin=[]  DivideOutMax=[]  UdiffTsProdOutMin=[]  UdiffTsProdOutMax=[]  NTsProdOutMin=[]  NTsProdOutMax=[]  UintegralTsProdOutMin=[]  UintegralTsProdOutMax=[]  UngainTsProdOutMin=[]  UngainTsProdOutMax=[]  IntegratorContinuousStateAttributes=''  IntegratorStateMustResolveToSignalObject=off  IntegratorRTWStateStorageClass=Auto  FilterContinuousStateAttributes=''  FilterStateMustResolveToSignalObject=off  FilterRTWStateStorageClass=Auto  ParallelPVariant=InternalParameters  IdealPVariant=Disabled  IVariant=InternalParameters  DVariant=InternalParameters  bVariant=InternalParameters  cVariant=InternalParameters  IntegratorVariant=Discrete  SatVariant=Disabled  AWVariant=Passthrough  PCopyVariant=Disabled  TRVariant=Disabled  FdbkBlocksVariant=Forward  IdealPFdbkVariant=Disabled  SatFdbkVariant=Disabled  DerivativeFilterVariant=ForwardEulerFilter  NVariant=InternalParameters  NCopyVariant=Disabled  FilterICVariant=InternalICsFilter  IntegratorICVariant=InternalICs  ExternalResetVariant=Disabled  TRSumVariant=Passthrough  SumFdbkVariant=Disabled  SumVariant=Sum_PID  TsampFilterVariant=InternalTs  TsampNgainVariant=Passthrough  TsampIntegralVariant=Passthrough
  mass : DataStoreRead  DataStoreName=Structural_data  DataStoreElements=Structural_data(1,1)
  p : DataStoreRead  DataStoreName=Plane_state_store  DataStoreElements=Plane_state_store(1,4)
  p,q,r,phi,theta,psi : DataStoreRead  DataStoreName=Plane_state_store  DataStoreElements=Plane_state_store(1,4:9)
  phi : DataStoreRead  DataStoreName=Plane_state_store  DataStoreElements=Plane_state_store(1,7)
  Out1 : Outport  VectorParamsAs1DForOutWhenUnconnected=off
  wires:
  PID Controller (2DOF)1/1 -> Out1/1
  MATLAB Function1/1(phi_d) -> PID Controller (2DOF)/1
  p/1 -> PID Controller (2DOF)1/2
  phi/1 -> PID Controller (2DOF)/2
  p,q,r,phi,theta,psi/1 -> MATLAB Function2/1(angular_state)
  MATLAB Function2/1(p_d) -> PID Controller (2DOF)1/1
  PID Controller (2DOF)/1 -> MATLAB Function2/2(phi_dot_d)
  a_y_d/1 -> MATLAB Function1/4(a_y_d)
  Data Store Read/1 -> MATLAB Function1/2(TT)
  mass/1 -> MATLAB Function1/3(mass)
  Digital Clock/1 -> MATLAB Function1/1(t)

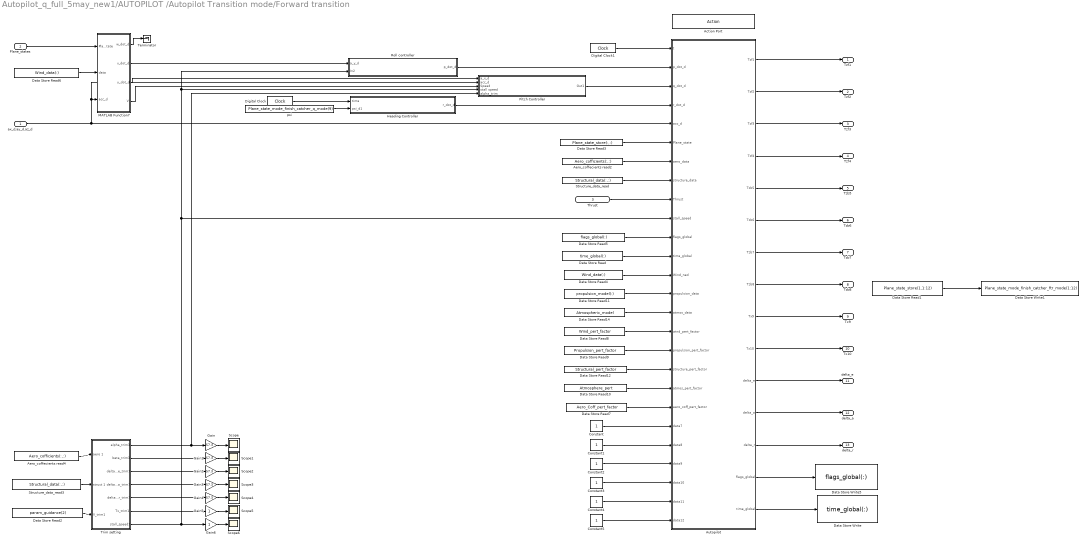
== system Autopilot_q_full_5may_new1/AUTOPILOT /Autopilot Transition mode/Forward transition ==
  ax_d,ay_d,az_d : Inport
  Plane_states : Inport  Port=2
  Thrust : Inport  Port=3
  Action Port : ActionPort  ActionPortLabel=if { }
  Aero_coffecients read2 : DataStoreRead  Priority=1  DataStoreName=Aero_cofficients  DataStoreElements=Aero_cofficients(:,:)
  Aero_coffecients read4 : DataStoreRead  DataStoreName=Aero_cofficients  DataStoreElements=Aero_cofficients(:,:)
  Autopilot : MATLAB Function  TreatAsAtomicUnit=on
  Constant{,1..5} (6 alike) : Constant
  Data Store Read : DataStoreRead  DataStoreName=time_global  DataStoreElements=time_global(:)
  Data Store Read1 : DataStoreRead  DataStoreName=Plane_state_store  DataStoreElements=Plane_state_store(1,1:12)
  Data Store Read10 : DataStoreRead  DataStoreName=Atmosphere_pert
  Data Store Read11 : DataStoreRead  DataStoreName=propulsion_model  DataStoreElements=propulsion_model(:)
  Data Store Read12 : DataStoreRead  DataStoreName=Structural_pert_factor
  Data Store Read14 : DataStoreRead  DataStoreName=Atmospheric_model
  Data Store Read2 : DataStoreRead  DataStoreName=param_guidance  DataStoreElements=param_guidance(2)
  Data Store Read3 : DataStoreRead  DataStoreName=Plane_state_store  DataStoreElements=Plane_state_store(:,:)
  Data Store Read4 : DataStoreRead  DataStoreName=Wind_data  DataStoreElements=Wind_data(:)
  Data Store Read5 : DataStoreRead  DataStoreName=flags_global  DataStoreElements=flags_global(:)
  Data Store Read6 : DataStoreRead  DataStoreName=Wind_data  DataStoreElements=Wind_data(:)
  Data Store Read7 : DataStoreRead  DataStoreName=Aero_Coff_pert_factor
  Data Store Read8 : DataStoreRead  DataStoreName=Wind_pert_factor
  Data Store Read9 : DataStoreRead  DataStoreName=Propulsion_pert_factor
  Data Store Write : DataStoreWrite  DataStoreName=time_global  DataStoreElements=time_global(:)
  Data Store Write1 : DataStoreWrite  DataStoreName=Plane_state_mode_finish_catcher_ftr_mode  DataStoreElements=Plane_state_mode_finish_catcher_ftr_mode(1:12)
  Data Store Write5 : DataStoreWrite  DataStoreName=flags_global  DataStoreElements=flags_global(:)
  Digital Clock : DigitalClock  SampleTime=0.01
  Digital Clock1 : DigitalClock  SampleTime=0.01
  Gain{,1..4} (5 alike) : Gain  Gain=57.3
  Gain5 : Gain
  Gain6 : Gain
  Heading Controller : Subsystem
  MATLAB Function7 : MATLAB Function  TreatAsAtomicUnit=on
  Pitch Controller : Subsystem
  Roll controller : Subsystem
  Scope{,1..6} (7 alike) : Scope
  Structure_data_read : DataStoreRead  Priority=2  DataStoreName=Structural_data  DataStoreElements=Structural_data(:,:)
  Structure_data_read3 : DataStoreRead  DataStoreName=Structural_data  DataStoreElements=Structural_data(:,:)
  Terminator : Terminator
  Trim setting : Subsystem
  psi : DataStoreRead  DataStoreName=Plane_state_mode_finish_catcher_q_mode  DataStoreElements=Plane_state_mode_finish_catcher_q_mode(9)
  Tzf1 : Outport  VectorParamsAs1DForOutWhenUnconnected=off
  Tzf2 : Outport  Port=2  VectorParamsAs1DForOutWhenUnconnected=off
  Tzf3 : Outport  Port=3  VectorParamsAs1DForOutWhenUnconnected=off
  Tzf4 : Outport  Port=4  VectorParamsAs1DForOutWhenUnconnected=off
  Tzb5 : Outport  Port=5  VectorParamsAs1DForOutWhenUnconnected=off
  Tzb6 : Outport  Port=6  VectorParamsAs1DForOutWhenUnconnected=off
  Tzb7 : Outport  Port=7  VectorParamsAs1DForOutWhenUnconnected=off
  Tzb8 : Outport  Port=8  VectorParamsAs1DForOutWhenUnconnected=off
  Tx9 : Outport  Port=9  VectorParamsAs1DForOutWhenUnconnected=off
  Tx10 : Outport  Port=10  VectorParamsAs1DForOutWhenUnconnected=off
  delta_e : Outport  Port=11  VectorParamsAs1DForOutWhenUnconnected=off
  delta_a : Outport  Port=12  VectorParamsAs1DForOutWhenUnconnected=off
  delta_r : Outport  Port=13  VectorParamsAs1DForOutWhenUnconnected=off
  wires:
  Autopilot/12(delta_a) -> delta_a/1
  Digital Clock/1 -> Heading Controller/1("time ")
  Autopilot/10(Tx10) -> Tx10/1
  Roll controller/1(p_dot_d) -> Autopilot/2(p_dot_d)
  Autopilot/4(Tzf4) -> Tzf4/1
  Autopilot/1(Tzf1) -> Tzf1/1
  Autopilot/8(Tzb8) -> Tzb8/1
  Heading Controller/1(r_dot_d) -> Autopilot/4(r_dot_d)
  Trim setting/1(alpha_trim1) -> Gain/1, Pitch Controller/5(alpha_trim)
  Autopilot/2(Tzf2) -> Tzf2/1
  Autopilot/5(Tzb5) -> Tzb5/1
  Autopilot/9(Tx9) -> Tx9/1
  Autopilot/11(delta_e) -> delta_e/1
  Autopilot/6(Tzb6) -> Tzb6/1
  Autopilot/3(Tzf3) -> Tzf3/1
  Autopilot/13(delta_r) -> delta_r/1
  Autopilot/7(Tzb7) -> Tzb7/1
  Trim setting/7(stall_speed1) -> Autopilot/10(stall_speed), Pitch Controller/4(stall speed), Roll controller/2(In2), Gain6/1
  Autopilot/14(flags_global) -> Data Store Write5/1
  Data Store Read5/1 -> Autopilot/11("flags_global ")
  Autopilot/15(time_global) -> Data Store Write/1
  Data Store Read/1 -> Autopilot/12("time_global ")
  Digital Clock1/1 -> Autopilot/1(t)
  Gain/1 -> Scope/1
  Gain1/1 -> Scope1/1
  Gain2/1 -> Scope2/1
  Gain3/1 -> Scope3/1
  Trim setting/5(delta_r_trim1) -> Gain4/1
  Gain4/1 -> Scope4/1
  Gain5/1 -> Scope5/1
  Trim setting/6(Tx_trim1) -> Gain5/1
  Gain6/1 -> Scope6/1
  Data Store Read1/1 -> Data Store Write1/1
  Pitch Controller/1(Out1) -> Autopilot/3(q_dot_d)
  ax_d,ay_d,az_d/1 -> MATLAB Function7/3(acc_d), Pitch Controller/2(acc_d), Autopilot/5(acc_d)
  psi/1 -> Heading Controller/2(psi_d1)
  Aero_coffecients read2/1 -> Autopilot/7(aero_data)
  Structure_data_read/1 -> Autopilot/8(structure_data)
  Thrust/1 -> Autopilot/9(Thrust)
  Plane_states/1 -> MATLAB Function7/1(Plane_state)
  MATLAB Function7/3(u_dot_d) -> Pitch Controller/1(a_x_d)
  MATLAB Function7/2(v_dot_d) -> Roll controller/1(a_y_d)
  MATLAB Function7/1(w_dot_d) -> Terminator/1
  MATLAB Function7/4(V) -> Pitch Controller/3(Speed)
  Data Store Read3/1 -> Autopilot/6(Plane_state)
  Data Store Read4/1 -> Autopilot/13(Wind_ned)
  Data Store Read6/1 -> MATLAB Function7/2(data)
  Data Store Read11/1 -> Autopilot/14(propulsion_data)
  Data Store Read14/1 -> Autopilot/15(atmos_data)
  Data Store Read8/1 -> Autopilot/16(wind_pert_factor)
  Data Store Read9/1 -> Autopilot/17(propulsion_pert_factor)
  Data Store Read12/1 -> Autopilot/18(structure_pert_factor)
  Data Store Read10/1 -> Autopilot/19(atmos_pert_factor)
  Data Store Read7/1 -> Autopilot/20(aero_coff_pert_factor)
  Constant/1 -> Autopilot/21(data7)
  Constant1/1 -> Autopilot/22(data8)
  Constant2/1 -> Autopilot/23(data9)
  Constant3/1 -> Autopilot/24(data10)
  Constant4/1 -> Autopilot/25(data11)
  Constant5/1 -> Autopilot/26(data12)
  Trim setting/2(beta_trim1) -> Gain1/1
  Trim setting/4(delta_a_trim1) -> Gain3/1
  Trim setting/3(delta_e_trim1) -> Gain2/1
  Aero_coffecients read4/1 -> Trim setting/1(aero 1)
  Structure_data_read3/1 -> Trim setting/2(struct 1)
  Data Store Read2/1 -> Trim setting/3(V_trim1)
